simulink model "twoPSK"  (R2018a)
settings: Solver=FixedStepAuto  StartTime=0.0  StopTime=20.0  FixedStep=1e-4  RelTol=1e-3
libraries: dsparch4 x2, commrandsrc3 x1
settings Model: Creator=mengmeng  LastModifiedBy=mengmeng

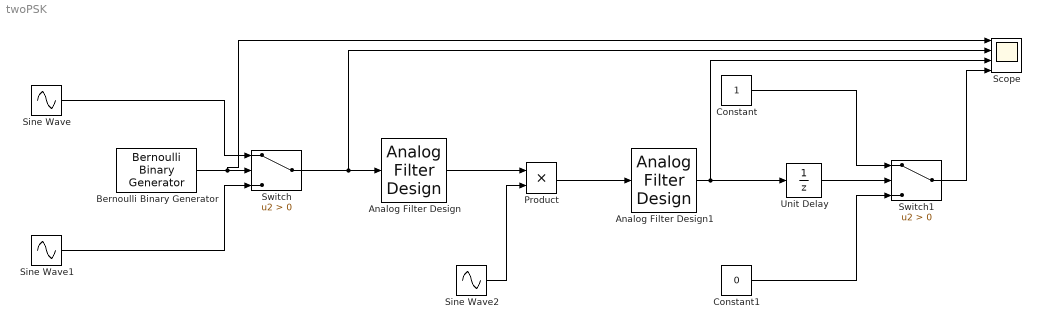
== system twoPSK ==
  Analog Filter Design : dsparch4/Analog Filter Design  method=Butterworth  filttype=Bandpass  N=8  Wlo=90  Whi=110  Rp=2  Rs=40
  Analog Filter Design1 : dsparch4/Analog Filter Design  method=Butterworth  filttype=Lowpass  N=8  Wlo=10  Whi=80  Rp=2  Rs=40
  Bernoulli Binary Generator : commrandsrc3/Bernoulli Binary Generator  ProbabilityOfZero=0.5  SeedSource=Parameter  Seed=61  SampleTime=1  SamplesPerFrame=1  OutputDataType=double  SimulateUsing=Interpreted execution
  Constant : Constant
  Constant1 : Constant  Value=0
  Product : Product
  Scope : Scope  NumInputPorts=4
  Sine Wave : Sin  Frequency=100  SampleTime=0
  Sine Wave1 : Sin  Frequency=100  Phase=pi  SampleTime=0
  Sine Wave2 : Sin  Frequency=100  SampleTime=0
  Switch : Switch  Criteria=u2 > Threshold
  Switch1 : Switch  Criteria=u2 > Threshold
  Unit Delay : UnitDelay  SampleTime=-1
  wires:
  Sine Wave/1 -> Switch/1
  Bernoulli Binary Generator/1 -> Scope/1, Switch/2
  Sine Wave1/1 -> Switch/3
  Switch/1 -> Scope/2, Analog Filter Design/1
  Analog Filter Design/1 -> Product/1
  Sine Wave2/1 -> Product/2
  Product/1 -> Analog Filter Design1/1
  Constant/1 -> Switch1/1
  Constant1/1 -> Switch1/3
  Analog Filter Design1/1 -> Scope/3, Unit Delay/1
  Unit Delay/1 -> Switch1/2
  Switch1/1 -> Scope/4
